simulink model "Lab1_parameter_estimation_student"  (R2025b)
settings: Solver=FixedStepAuto  StartTime=0.0  StopTime=20  FixedStep=0.0005  RelTol=1e-3
values from neighbouring files (symbols this model uses):
  motor_B = 0.00000214    (= 2.14e-06)    [Lab1_motor_params_student.m]
  motor_Eff = 0.9784300    (= 0.97843)    [Lab1_motor_params_student.m]
  motor_J = 0.000011739    (= 1.1739e-05)    [Lab1_motor_params_student.m]
  motor_Ke = 0.050668    [Lab1_motor_params_student.m]
  motor_L = 0.003313    [Lab1_motor_params_student.m]
  motor_R = 3.57    [Lab1_motor_params_student.m]
libraries: simulink x5, eeStairGenerator x4
settings Model: Creator=tanawatp  LastModifiedBy=Akkarasaknarong
settings RTWCC: GPUComputeCapability=3.5

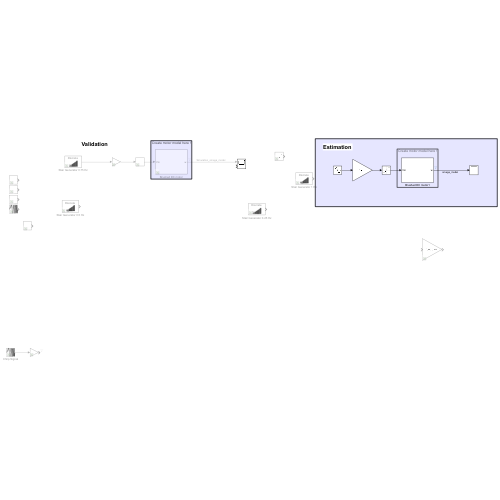
[thumbnail: Simulink's stored preview of the top-level diagram]
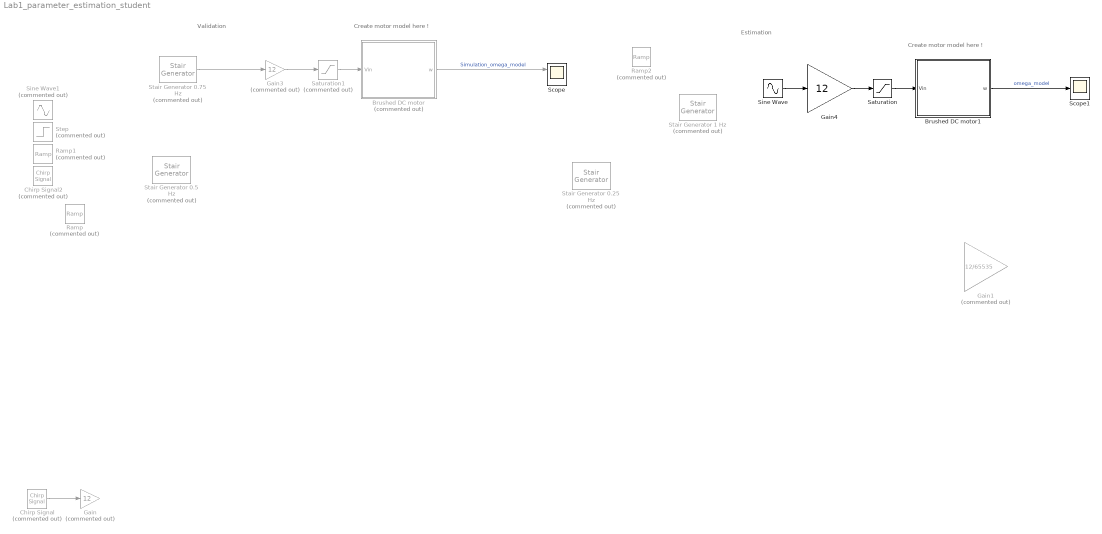
== system Lab1_parameter_estimation_student ==
  note: Validation
  note: Estimation
  note: Create motor model here !
  note: Create motor model here !
  Brushed DC motor : Subsystem  Commented=on
  Brushed DC motor1 : Subsystem
  Chirp Signal : simulink/Sources/Chirp Signal  Commented=on  f1=0.1  T=40  f2=5
  Chirp Signal2 : simulink/Sources/Chirp Signal  Commented=on  f1=0  T=35  f2=2
  Gain : Gain  Commented=on  Gain=12
  Gain1 : Gain  Commented=on  Gain=12/65535
  Gain3 : Gain  Commented=on  Gain=12
  Gain4 : Gain  Gain=12
  Ramp : simulink/Sources/Ramp  Commented=on  slope=0.25  start=2  InitialOutput=0
  Ramp1 : simulink/Sources/Ramp  Commented=on  slope=0.15  start=2  InitialOutput=0
  Ramp2 : simulink/Sources/Ramp  Commented=on  slope=0.25  start=2  InitialOutput=0
  Saturation : Saturate  UpperLimit=12  LowerLimit=-12
  Saturation1 : Saturate  Commented=on  UpperLimit=12  LowerLimit=-12
  Scope : Scope  NumInputPorts=2
      settings: ActiveDisplayYMinimum=-8191.8749999999982  ActiveDisplayYMaximum=73726.875
  Scope1 : Scope
      settings: ActiveDisplayYMinimum=-34.239482473644017  ActiveDisplayYMaximum=51.071650378806922
  Sine Wave : Sin  Frequency=1*2*pi  SampleTime=0
  Sine Wave1 : Sin  Commented=on  Frequency=0.5*2*pi  SampleTime=0
  Stair Generator 0.25 Hz : eeStairGenerator/Stair Generator  Commented=on  LabelModeActiveChoice=Discrete  TimeInput=[0.25 0.5 0.75 1 1.25 1.5 1.75 2 2.25 2.5 2.75 3 3.25 3.5 3.75 4 4.25 4.5 4.75 5]  AmplitudeInput=[0 0.1 0 0.2 0 0.3 0 0.4 0 0.5 0 0.6 0 0.7 0 0.8 0 0.9 0 1]  SampleTime=0.0002  RepeatPattern=off  OutDataTypeStr=double
      settings: LibrarySourceBlock=ee_sl_lib/General Control/Stair Generator
  Stair Generator 0.5 Hz : eeStairGenerator/Stair Generator  Commented=on  LabelModeActiveChoice=Discrete  TimeInput=[0.5 1 1.5 2 2.5 3 3.5 4 4.5 5 5.5 6 6.5 7 7.5 8 8.5 9 9.5 10]  AmplitudeInput=[0 0.1 0 0.2 0 0.3 0 0.4 0 0.5 0 0.6 0 0.7 0 0.8 0 0.9 0 1]  SampleTime=0.0002  RepeatPattern=off  OutDataTypeStr=double
      settings: LibrarySourceBlock=ee_sl_lib/General Control/Stair Generator
  Stair Generator 0.75 Hz : eeStairGenerator/Stair Generator  Commented=on  LabelModeActiveChoice=Discrete  TimeInput=[0.75 1.5 2.25 3 3.75 4.5 5.25 6 6.75 7.5 8.25 9 9.75 10.5 11.25 12 12.75 13.5 14.25 15]  AmplitudeInput=[0 0.1 0 0.2 0 0.3 0 0.4 0 0.5 0 0.6 0 0.7 0 0.8 0 0.9 0 1]  SampleTime=0.0002  RepeatPattern=off  OutDataTypeStr=double
      settings: LibrarySourceBlock=ee_sl_lib/General Control/Stair Generator
  Stair Generator 1 Hz : eeStairGenerator/Stair Generator  Commented=on  LabelModeActiveChoice=Discrete  TimeInput=[1 2 3 4 5 6 7 8 9 10 11 12 13 14 15 16 17 18 19 20]  AmplitudeInput=[0 0.1 0 0.2 0 0.3 0 0.4 0 0.5 0 0.6 0 0.7 0 0.8 0 0.9 0 1]  SampleTime=0.0002  RepeatPattern=off  OutDataTypeStr=double
      settings: LibrarySourceBlock=ee_sl_lib/General Control/Stair Generator
  Step : Step  Commented=on  Time=10  After=0.6*12  SampleTime=0
  wires:
  Brushed DC motor/1(w) -> Scope/1  "Simulation_omega_model"
  Chirp Signal/1 -> Gain/1
  Sine Wave/1 -> Gain4/1
  Saturation1/1 -> Brushed DC motor/1(Vin)
  Gain4/1 -> Saturation/1
  Brushed DC motor1/1(w) -> Scope1/1  "omega_model"
  Stair Generator 0.75 Hz/1 -> Gain3/1
  Gain3/1 -> Saturation1/1
  Saturation/1 -> Brushed DC motor1/1(Vin)

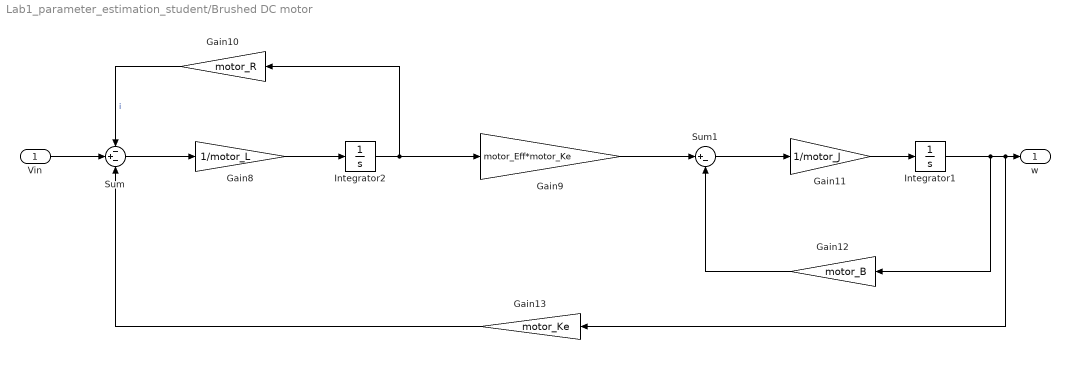
== system Lab1_parameter_estimation_student/Brushed DC motor ==
  Vin : Inport
  Gain10 : Gain  Gain=motor_R
  Gain11 : Gain  Gain=1/motor_J
  Gain12 : Gain  Gain=motor_B
  Gain13 : Gain  Gain=motor_Ke
  Gain8 : Gain  Gain=1/motor_L
  Gain9 : Gain  Gain=motor_Eff*motor_Ke
  Integrator1 : Integrator
  Integrator2 : Integrator
  Sum : Sum  Inputs=-+-
  Sum1 : Sum  Inputs=|+-
  w : Outport
  wires:
  Sum/1 -> Gain8/1
  Gain8/1 -> Integrator2/1
  Integrator2/1 -> Gain9/1, Gain10/1
  Gain10/1 -> Sum/1  "i"
  Vin/1 -> Sum/2
  Gain9/1 -> Sum1/1
  Sum1/1 -> Gain11/1
  Gain11/1 -> Integrator1/1
  Integrator1/1 -> Gain12/1, Gain13/1, w/1
  Gain13/1 -> Sum/3
  Gain12/1 -> Sum1/2

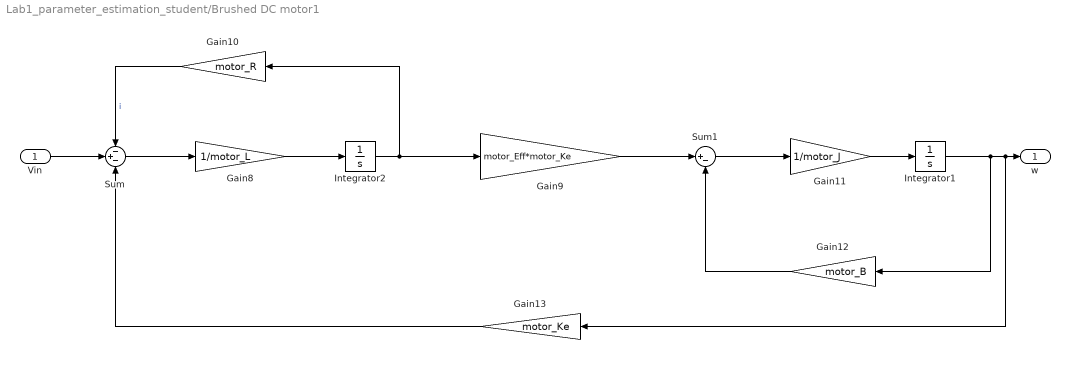
== system Lab1_parameter_estimation_student/Brushed DC motor1 ==
  Vin : Inport
  Gain10 : Gain  Gain=motor_R
  Gain11 : Gain  Gain=1/motor_J
  Gain12 : Gain  Gain=motor_B
  Gain13 : Gain  Gain=motor_Ke
  Gain8 : Gain  Gain=1/motor_L
  Gain9 : Gain  Gain=motor_Eff*motor_Ke
  Integrator1 : Integrator
  Integrator2 : Integrator
  Sum : Sum  Inputs=-+-
  Sum1 : Sum  Inputs=|+-
  w : Outport
  wires:
  Sum/1 -> Gain8/1
  Gain8/1 -> Integrator2/1
  Integrator2/1 -> Gain9/1, Gain10/1
  Gain10/1 -> Sum/1  "i"
  Vin/1 -> Sum/2
  Gain9/1 -> Sum1/1
  Sum1/1 -> Gain11/1
  Gain11/1 -> Integrator1/1
  Integrator1/1 -> Gain12/1, Gain13/1, w/1
  Gain13/1 -> Sum/3
  Gain12/1 -> Sum1/2
